simulink model "New_Wing_Monocopter_Testing"  (R2022b)
settings: Solver=ode23t  StartTime=0.0  StopTime=50  MaxStep=1e-3  RelTol=1e-3  AbsTol=1e-3
values from neighbouring files (symbols this model uses):
  air_rho = 1.225    [inherited_params.mat]
  battery_capacity = 22.8    [inherited_params.mat]
  CDO = 0.155    [inherited_params.mat]
  filtD_motor = 10000    [inherited_params.mat]
  filtSpd_motor = 0.001    [inherited_params.mat]
  kd_motor = 0    [inherited_params.mat]
  ki_motor = 0.00045    [inherited_params.mat]
  limit_motor = 0.25    [inherited_params.mat]
  monoco_mass = 0.16    [inherited_params.mat]
  monoco_prop =     [inherited_params.mat]
  monoco_radius = 0.57913    [inherited_params.mat]
  monoco_wing =     [inherited_params.mat]
  monoco_wing_area = 0.05668053    [inherited_params.mat]
  waypoints = [-2 -2 0.14 -2 -2 6 0 0 6 2 0 6 ... (15 elements, 3x5)]    [inherited_params.mat]
undefined symbols (not defined in the file or in its folder): drag_linear, drag_quad, flap_radius, flap_surface_area, klinear, kquad, X, Y, Z
libraries: sm_lib x96, nesl_utility x38, slpidlib x18, fl_lib x12, sdl_lib x3, simulink x2, simulink_extras x1, batteryecm_lib x1, ee_lib x1
(part 6 of 6)

== system New_Wing_Monocopter_Testing/Monowing/Monowing_Assem/Flap control ==
  y : Inport
  Conversion to deg : Gain  Gain=180/pi
  Conversion to rad : Gain  Gain=pi/180
  File Solid : sm_lib/Body Elements/File Solid  ExtGeomFileName=C:\Users\emman\Monocopter_Frame\DmMc_Wing_type7_Flap2.STEP  UnitType=FromFile  ExtGeomFileUnits=m  StepReaderType=HEX  ExportConvexHullGeometry=off  InertiaType=CalculateFromGeometry  Mass=0.57  MassUnits=g  CenterOfMass=[0 0 0]  CenterOfMassUnits=m  MomentsOfInertia=[1 1 1]  MomentsOfInertiaUnits=kg*m^2  ProductsOfInertia=[0 0 0]  ProductsOfInertiaUnits=kg*m^2  BasedOnType=Mass  Density=1000  DensityUnits=kg/m^3  DoExposeReferenceFrame=off  SerializedFrames=<Frames><Frame><Id>Frame1</Id><Value><Name>Flap_hinge</Name><Origin><Source>GeometricFeature</Source><FeatureName>planar surface 5</FeatureName></Origin><PrimaryAxis><DefinedDirection>+Z</DefinedDirection><Source>GeometricFeature</Source><SourceDirection>+Z</SourceDirection><FeatureName>segment 10</FeatureName></PrimaryAxis><SecondaryAxis><DefinedDirection>+X</DefinedDirection><Source>ReferenceFrame</Source><SourceDirection>+X</SourceDirection><FeatureName></FeatureName></SecondaryAxis></Value></Frame><Frame><Id>Frame2</Id><Value><Name>Flap_contact_1</Name><Origin><Source>GeometricFeature</Source><FeatureName>point 5</FeatureName></Origin><PrimaryAxis><DefinedDirection>+Z</DefinedDirection><Source>ReferenceFrame</Source><SourceDirection>+Z</SourceDirection><FeatureName></FeatureName></PrimaryAxis><SecondaryAxis><DefinedDirection>+X</DefinedDirection><Source>ReferenceFrame</Source><SourceDirection>+X</SourceDirection><FeatureName></FeatureName></SecondaryAxis></Value></Frame><Frame><Id>Frame3</Id><Value><Name>Flap_contact_2</Name><Origin><Source>GeometricFeature</Source><FeatureName>point 7</FeatureName></Origin><PrimaryAxis><DefinedDirection>+Z</DefinedDirection><Source>ReferenceFrame</Source><SourceDirection>+Z</SourceDirection><FeatureName></FeatureName></PrimaryAxis><SecondaryAxis><DefinedDirection>+X</DefinedDirection><Source>ReferenceFrame</Source><SourceDirection>+X</SourceDirection><FeatureName></FeatureName></SecondaryAxis></Value></Frame><Frame><Id>Frame4</Id><Value><Name>Flap_Moment</Name><Origin><Source>CenterOfMassFrame</Source><FeatureName></FeatureName></Origin><PrimaryAxis><DefinedDirection>+Z</DefinedDirection><Source>ReferenceFrame</Source><SourceDirection>+Z</SourceDirection><FeatureName></FeatureName></PrimaryAxis><SecondaryAxis><DefinedDirection>+X</DefinedDirection><Source>ReferenceFrame</Source><SourceDirection>+X</SourceDirection><FeatureName></FeatureName></SecondaryAxis></Value></Frame></Frames>  GraphicType=FromGeometry  MarkerShape=Sphere  MarkerSize=10  GraphicVisPropType=SimpleVisualProperties  GraphicDiffuseColor=[0.5 0.5 0.5]  GraphicSpecularColor=[0.5 0.5 0.5 1.0]  GraphicAmbientColor=[0.15 0.15 0.15 1.0]  GraphicEmissiveColor=[0.0 0.0 0.0 1.0]  GraphicShininess=75  GraphicOpacity=1.0
  PS-Simulink Converter : nesl_utility/PS-Simulink Converter  PhysicalDomain=network_engine_domain  SubClassName=ps_output  LeftPortType=input  RightPortType=output  PseudoPeriodic=off  Frequencies=[]  VectorFormat=inherit  Unit=inherit  AffineConversion=off
  Revolute Joint : sm_lib/Joints/Revolute Joint  JointMode=Normal  SenseConstraintForce=off  SenseConstraintForceX=off  SenseConstraintForceY=off  SenseConstraintForceZ=off  SenseConstraintTorque=off  SenseConstraintTorqueX=off  SenseConstraintTorqueY=off  SenseConstraintTorqueZ=off  SenseTotalForce=off  SenseTotalForceX=off  SenseTotalForceY=off  SenseTotalForceZ=off  SenseTotalTorque=off  SenseTotalTorqueX=off  SenseTotalTorqueY=off  SenseTotalTorqueZ=off  CompositeWrenchDir=FollowerOnBase  CompositeWrenchFrame=BaseFrame  EquilibriumPosition=0  EquilibriumPositionUnits=rad  SpringStiffness=0  SpringStiffnessUnits=N*m/deg  DampingCoefficient=0  DampingCoefficientUnits=N*m/(deg/s)  TorqueActuationMode=ComputedTorque  MotionActuationMode=InputMotion  SensePosition=on  SenseVelocity=off  SenseAcceleration=off  SenseTorqueForce=off  SenseLowerLimitTorqueForce=off  SenseUpperLimitTorqueForce=off  LowerLimitSpecify=off  LowerLimitBound=-20  LowerLimitBoundUnits=deg  LowerLimitStiffness=1e4  LowerLimitStiffnessUnits=N*m/deg  LowerLimitDamping=10  LowerLimitDampingUnits=N*m/(deg/s)  LowerLimitTransitionRegionWidth=0.1  LowerLimitTransitionRegionWidthUnits=deg  UpperLimitSpecify=off  UpperLimitBound=0  UpperLimitBoundUnits=deg  UpperLimitStiffness=1e4  UpperLimitStiffnessUnits=N*m/deg  UpperLimitDamping=10  UpperLimitDampingUnits=N*m/(deg/s)  UpperLimitTransitionRegionWidth=0.1  UpperLimitTransitionRegionWidthUnits=deg  PositionTargetSpecify=on  PositionTargetPriority=High  PositionTargetValue=0.0  PositionTargetValueUnits=rad  VelocityTargetSpecify=off  VelocityTargetPriority=High  VelocityTargetValue=0  VelocityTargetValueUnits=deg/s
  Rigid Transform9 : sm_lib/Frames and Transforms/Rigid Transform  TranslationMethod=Cartesian  TranslationStandardOffset=0  TranslationLengthUnit=mm  TranslationStandardAxis=+Z  TranslationCartesianOffset=[-1.5 -0.25 0.2]  TranslationROffset=0  TranslationROffsetUnits=m  TranslationZOffset=0  TranslationZOffsetUnits=m  TranslationThetaOffset=0  TranslationThetaOffsetUnits=deg  RotationMethod=None  RotationAngleUnits=deg  RotationStandardAxis=+Z  RotationAngle=0.0  RotationArbitraryAxis=[0 0 1]  FollAlignAxisA=+X  BaseAlignAxisA=+Y  FollAlignAxisB=+Y  BaseAlignAxisB=+Z  RotationSequenceAxes=FollowerAxes  RotationSequence=XYX  RotationSequenceAngles=[0 0 0]  RotationSequenceAnglesUnits=deg  RotationMatrix=[1 0 0; 0 1 0; 0 0 1]  Quaternion=[1 0 0 0]
  Simulink-PS Converter : nesl_utility/Simulink-PS Converter  PhysicalDomain=network_engine_domain  SubClassName=ps_input  LeftPortType=input  RightPortType=output  PseudoPeriodic=off  Frequencies=[]  NoiseDistribution=none  NoiseParameters=[]  Unit=rad  AffineConversion=off  FilteringAndDerivatives=filter  SimscapeFilterOrder=2  InputFilterTimeConstant=0.01  UdotUserProvided=0
  Transfer Fcn (with initial outputs) : simulink_extras/Additional Linear/Transfer Fcn (with initial outputs)  N=[1]  D="[0.01  1]"  Y0=.5  U0=0
  Conn1 : PMIOPort  Side=Left
  Flap Contact 1 : PMIOPort  Port=2  Side=Left
  Flap Contact 2 : PMIOPort  Port=3  Side=Left
  Flap Moment : PMIOPort  Port=4  Side=Left
  Out1 : Outport
  wires:
  Conversion to rad/1 -> Transfer Fcn (with initial outputs)/1
  Transfer Fcn (with initial outputs)/1 -> Simulink-PS Converter/1
  PS-Simulink Converter/1 -> Conversion to deg/1
  y/1 -> Conversion to rad/1
  Conversion to deg/1 -> Out1/1
  connections:
  Revolute Joint/RConn1 -- File Solid/LConn1
  Revolute Joint/LConn1 -- Rigid Transform9/RConn1
  Simulink-PS Converter/RConn1 -- Revolute Joint/LConn2
  PS-Simulink Converter/LConn1 -- Revolute Joint/RConn2
  Rigid Transform9/LConn1 -- Conn1/RConn1
  File Solid/RConn1 -- Flap Contact 1/RConn1
  Flap Contact 2/RConn1 -- File Solid/LConn2
  Flap Moment/RConn1 -- File Solid/RConn2

== system New_Wing_Monocopter_Testing/Collective Control/PD Alt Controller (Monoco negative direction counter clockwise)/Low Pass Filter/If Action Subsystem ==
  In1 : Inport
  Action Port : ActionPort  ActionPortLabel=else
  Out1 : Outport
  wires:
  In1/1 -> Out1/1

== system New_Wing_Monocopter_Testing/Collective Control/PD Alt Controller (Monoco negative direction counter clockwise)/Low Pass Filter/If Action Subsystem1 ==
  In1 : Inport
  Action Port : ActionPort  ActionPortLabel=if(u1<(-2200))
  Out1 : Outport
  wires:
  In1/1 -> Out1/1

== system New_Wing_Monocopter_Testing/Collective Control/PD Alt Controller (Monoco positve direction clockwise)/Low Pass Filter/If Action Subsystem ==
  In1 : Inport
  Action Port : ActionPort  ActionPortLabel=else
  Out1 : Outport
  wires:
  In1/1 -> Out1/1

== system New_Wing_Monocopter_Testing/Collective Control/PD Alt Controller (Monoco positve direction clockwise)/Low Pass Filter/If Action Subsystem1 ==
  In1 : Inport
  Action Port : ActionPort  ActionPortLabel=if(u1>(2300))
  Out1 : Outport
  wires:
  In1/1 -> Out1/1

== system New_Wing_Monocopter_Testing/Cyclic Roll Control/PD Pitch Controller (Monoco negative direction counter clockwise) Back Motor/Low Pass Filter/If Action Subsystem ==
  In1 : Inport
  Action Port : ActionPort
  Out1 : Outport
  wires:
  In1/1 -> Out1/1

== system New_Wing_Monocopter_Testing/Cyclic Roll Control/PD Pitch Controller (Monoco negative direction counter clockwise) Back Motor/Low Pass Filter/If Action Subsystem1 ==
  In1 : Inport
  Action Port : ActionPort
  Out1 : Outport
  wires:
  In1/1 -> Out1/1

== system New_Wing_Monocopter_Testing/Cyclic Roll Control/PD Pitch Controller (Monoco negative direction counter clockwise) Front Motor/Low Pass Filter/If Action Subsystem ==
  In1 : Inport
  Action Port : ActionPort
  Out1 : Outport
  wires:
  In1/1 -> Out1/1

== system New_Wing_Monocopter_Testing/Cyclic Roll Control/PD Pitch Controller (Monoco negative direction counter clockwise) Front Motor/Low Pass Filter/If Action Subsystem1 ==
  In1 : Inport
  Action Port : ActionPort
  Out1 : Outport
  wires:
  In1/1 -> Out1/1

== system New_Wing_Monocopter_Testing/Cyclic Roll Control/PD Pitch Controller (Monoco negative direction counter clockwise)2/Low Pass Filter/If Action Subsystem ==
  In1 : Inport
  Action Port : ActionPort
  Out1 : Outport
  wires:
  In1/1 -> Out1/1

== system New_Wing_Monocopter_Testing/Cyclic Roll Control/PD Pitch Controller (Monoco negative direction counter clockwise)2/Low Pass Filter/If Action Subsystem1 ==
  In1 : Inport
  Action Port : ActionPort
  Out1 : Outport
  wires:
  In1/1 -> Out1/1

== system New_Wing_Monocopter_Testing/Cyclic Roll Control/PD Roll Controller (Monoco negative direction counter clockwise) Back Motor/Low Pass Filter/If Action Subsystem ==
  In1 : Inport
  Action Port : ActionPort
  Out1 : Outport
  wires:
  In1/1 -> Out1/1

== system New_Wing_Monocopter_Testing/Cyclic Roll Control/PD Roll Controller (Monoco negative direction counter clockwise) Back Motor/Low Pass Filter/If Action Subsystem1 ==
  In1 : Inport
  Action Port : ActionPort
  Out1 : Outport
  wires:
  In1/1 -> Out1/1

== system New_Wing_Monocopter_Testing/Cyclic Roll Control/PD Roll Controller (Monoco negative direction counter clockwise) Front Motor/Low Pass Filter/If Action Subsystem ==
  In1 : Inport
  Action Port : ActionPort
  Out1 : Outport
  wires:
  In1/1 -> Out1/1

== system New_Wing_Monocopter_Testing/Cyclic Roll Control/PD Roll Controller (Monoco negative direction counter clockwise) Front Motor/Low Pass Filter/If Action Subsystem1 ==
  In1 : Inport
  Action Port : ActionPort
  Out1 : Outport
  wires:
  In1/1 -> Out1/1

== matlab function New_Wing_Monocopter_Testing/Monowing/Speed Brake mode/Speed Brake Mode Activation ==
  data: rps input; y output; monoco_radius parameter; pitch input; air_rho parameter; monoco_wing_area parameter; Time input; Mode input
function y = fcn(rps, monoco_radius, pitch, air_rho, monoco_wing_area, Time, Mode)
linear_vel_sq = zeros(1,1);
linear_vel_sq = (rps * monoco_radius)^2;
drag_angle = 120;
drag_coeff = 0.1;



if Mode == 0
    if (pitch > drag_angle) && (Time < 8.0) 
        y = 0.5 * drag_coeff * air_rho * monoco_wing_area * linear_vel_sq * monoco_radius;
    else
        y = 0.0;
    end
else
    y = 0.0;
end

== matlab function New_Wing_Monocopter_Testing/Monowing/Collective Control/Collective (Anhedral) ==
  data: Torque_negative input; Toggle input; output output
function output  = fcn(Torque_negative, Toggle)

if Toggle == 2.0
    output = Torque_negative * 1.0; % change this 
else
    output = 0.0;
end
%y = Torque_negative;

== matlab function New_Wing_Monocopter_Testing/Monowing/Drag State/Drag filter ==
  data: drag input; Time input; drag_upper output; drag_lower output; Mode input
function [drag_upper, drag_lower] = fcn(drag, Time, Mode)
if Mode == 0
    if Time > 8.0 && Time < 12.0
        drag_upper = drag;
        drag_lower = 0.0;
    elseif Time > 12.0
        drag_lower = -1 * drag;
        drag_upper = 0.0;
    else
        drag_upper = drag;
        drag_lower = 0.0;
    end

elseif Mode == 1
    drag_upper = drag;
    drag_lower = 0.0;

else
    drag_upper = 0.0;
    drag_lower = -1 * drag;

end

== matlab function New_Wing_Monocopter_Testing/Hover ==
  data: Y output; toggle_y output; X output; toggle_x output; Time input
function [Y, toggle_y, X, toggle_x] = fcn(Time)

sol_X = zeros(1,1);
sol_Toggle_Y = zeros(1,1);
sol_Toggle_X = zeros(1,1);
sol_Y = zeros(1,1);
Velocity = 0.2;

if Time > 10 && Time < 40
%     if Time > 10 && Time < 15
%         sol_X = 0;
%         sol_Toggle_Y = 1;
%         sol_Toggle_X = 1;
%         sol_Y = -1;
%     
%     elseif Time > 15 && Time < 20
%         sol_X = 0;
%         sol_Toggle_Y = 1;
%         sol_Toggle_X = 1;
%         sol_Y = 0;
%     
%     elseif Time > 20 && Time < 25
%         sol_X = 0;
%         sol_Toggle_Y = 1;
%         sol_Toggle_X = 1;
%         sol_Y = 1;
% 
%     elseif Time > 25 && Time < 30
%         sol_X = 0;
%         sol_Toggle_Y = 1;
%         sol_Toggle_X = 1;
%         sol_Y = 0;
%     end
% 
% else
    sol_X = 0;
    sol_Y = 0;
    sol_Toggle_Y = 1;
    sol_Toggle_X = 1;
end

Y = sol_Y;
X = sol_X;
toggle_y = sol_Toggle_Y;
toggle_x = sol_Toggle_X;

== matlab function New_Wing_Monocopter_Testing/Monowing/Monowing_Assem/Collective & Cyclic Command Distribution (Dihedral Pitch) abt Yw ==
  data: u input; flap_dihedral_pitch_cmd output; gain_x input; heading input; Toggle input; Motor_Pulse output
function [flap_dihedral_pitch_cmd,Motor_Pulse] = fcn(u, gain_x, heading, Toggle)

if Toggle == 1 % Front Motor

    azimuth = u;
    if (abs(azimuth) > pi/4) && (abs(azimuth) < 3*pi/4)
        tilt_xw = sin(azimuth + heading); % tilt about yw heading in x direction 
        pitch = zeros(1,1);
        pitch = tilt_xw * gain_x; % only for cyclic y
        Motor_Pulse =  (pitch/abs(pitch)) * 1;

        if abs(pitch) > 0.75
            pitch = (pitch/abs(pitch)) * 0.75;
        end

        flap_dihedral_pitch_cmd = pitch;

    else
        
        Motor_Pulse =  0;
        flap_dihedral_pitch_cmd = 0.0;

    end

elseif Toggle == 2 % Back Motor

    azimuth = u;
    if (abs(azimuth) > pi/4) && (abs(azimuth) < 3*pi/4)
        tilt_xw = sin(azimuth + heading); % tilt around xw heading in y direction 
        pitch = zeros(1,1);
        pitch = tilt_xw * gain_x; % only for cyclic y
        Motor_Pulse =  (pitch/abs(pitch)) * 1;

        if abs(pitch) > 0.75
            pitch = (pitch/abs(pitch)) * 0.75;
        end

        flap_dihedral_pitch_cmd = pitch;

    else
        
        Motor_Pulse =  0;
        flap_dihedral_pitch_cmd = 0.0;

    end

else
    
    Motor_Pulse =  0;
    flap_dihedral_pitch_cmd = 0.0;

end





% kp = 1.3;
% desired_roll = 10;
% if (Annular_roll/abs(Annular_roll)) > 0.0
%     error_gain = kp*(Annular_roll - desired_roll);
% 
% elseif (Annular_roll/abs(Annular_roll)) < 0.0
%     error_gain = kp*(Annular_roll - (-1*desired_roll));
% 
% else
%     error_gain = 0.0;
% 
% end

% roll = gain * desired_flap * 2; % only for cyclic (original) 
% roll = desired_flap; % collective
% flap_cmd = roll - error_gain;

== matlab function New_Wing_Monocopter_Testing/Monowing/Monowing_Assem/Cyclic Command Distribution ==
  data: pitch_gain_dihedral_front input; roll_gain_dihedral_front input; pitch_gain_dihedral_back input; roll_gain_dihedral_back input; Transition_Mode output; gain_x output; gain_y output; Dihedral_Mode output; Mode_Selection input
function [Transition_Mode, gain_x, gain_y, Dihedral_Mode] = fcn(pitch_gain_dihedral_front, roll_gain_dihedral_front, pitch_gain_dihedral_back, roll_gain_dihedral_back, Mode_Selection)

if Mode_Selection == 1
    Transition_Mode = 0;
    Dihedral_Mode = 1;
    gain_x = pitch_gain_dihedral_front;
    gain_y = roll_gain_dihedral_front;
else 
    Transition_Mode = 0;
    Dihedral_Mode = 2;
    gain_x = pitch_gain_dihedral_back;
    gain_y = roll_gain_dihedral_back;
end



% if Mode_Selection == 0
%     Transition_Mode = 1;
%     Dihedral_Mode = 0;
%     Anhedral_Mode = 0;
%     gain_x = 0;
%     gain_y = 0;
% elseif Mode_Selection == 1
%     Transition_Mode = 0;
%     Dihedral_Mode = 1;
%     Anhedral_Mode = 0;
%     gain_x = pitch_gain_dihedral;
%     gain_y = roll_gain_dihedral;
% elseif Mode_Selection == 2
%     Transition_Mode = 0;
%     Dihedral_Mode = 0;
%     Anhedral_Mode = 1;
%     gain_x = pitch_gain_anhedral;
%     gain_y = roll_gain_anhedral;
% else 
%     Transition_Mode = 0;
%     Dihedral_Mode = 0;
%     Anhedral_Mode = 0;
%     gain_x = 0;
%     gain_y = 0;
% end

== matlab function New_Wing_Monocopter_Testing/Monowing/Collective Control/Collective Mode Switcher ==
  data: dihedral output; Time input; anhedral output; Mode input
function [dihedral,anhedral] = fcn(Time,Mode)
if Mode == 1
      dihedral = 1.0;
      anhedral = 0.0;
    
elseif Mode == 2
    dihedral = 1.0;
    anhedral = 0.0;
else
    dihedral = 0.0;
    anhedral = 0.0;
end


% if Mode == 0
%     
%     if Time > 8.0 && Time < 12.0
%         dihedral = 0.0; % upside cut torque
%         anhedral = 0.0;
%     elseif Time > 10
%         dihedral = 0.0;
%         anhedral = 1.0;
%     else
%         dihedral = 1.0;
%         anhedral = 0.0;
%     end
% 
% elseif Mode == 1
% 
%     dihedral = 1.0;
%     anhedral = 0.0;
% 
% elseif Mode == 2
% 
%     dihedral = 0.0;
%     anhedral = 1.0;
% 
% else
% 
%     dihedral = 0.0;
%     anhedral = 0.0;
% 
% end

== matlab function New_Wing_Monocopter_Testing/Monowing/Horizontal Forces/Horizontal Motion X ==
  data: roll_in_deg input; force output; Lift input; flap_angle_data input; vx input; vy input; vz input; klinear parameter; kquad parameter; pos_x input; azimuth input; flap_angle input
function force  = fcn(roll_in_deg, Lift, flap_angle_data, vx, vy, vz, klinear, kquad, pos_x, azimuth, flap_angle)
fx = zeros(1,1);
x = zeros(1,1);
v_l1 = zeros(1,1);
v_l2 = zeros(1,1);
roll_angle = abs(roll_in_deg);
%disp(Lift);
dihedral_offset = 2.0;
v_l1 = abs(vx) + abs(vy) + abs(vz);
v_l2 = sqrt(vx^2 + vy^2 + vz^2);

negative_x = 0;
positive_x = 1;
neutral_x = 2;

if azimuth > 0 && flap_angle > 0 
    current_state = negative_x;
    
elseif azimuth < 0 && flap_angle < 0
    current_state = negative_x;

elseif azimuth > 0 && flap_angle < 0
    current_state = positive_x;

elseif azimuth < 0 && flap_angle > 0
    current_state = positive_x;

else
    current_state = neutral_x;
end

%disp (current_state);
% disp (azimuth);
% disp (flap_angle);

% current_state = negative_y;

switch(current_state)

    case negative_x
        if roll_in_deg > 0 && roll_in_deg > dihedral_offset 
        %     if roll_in_deg > 0
            fx = Lift*sind(roll_in_deg-dihedral_offset);
            x = (-1*fx) + (kquad*v_l1*abs(vy) + klinear*abs(vy));
        elseif roll_in_deg < 0
            fx = Lift*sind(roll_angle);
            x = (-1*fx) + (kquad*v_l1*abs(vy) + klinear*abs(vy));
            %y = y  (kquad*v_l1*abs(vy) + klinear*abs(vy));
        else
            x = 0.0;
        end

    case positive_x
        if roll_in_deg > 0 && roll_in_deg > dihedral_offset 
        %     if roll_in_deg > 0
            fx = Lift*sind(roll_in_deg-dihedral_offset);
            x = fx - (kquad*v_l1*abs(vy) + klinear*abs(vy));
        elseif roll_in_deg < 0
            fx = Lift*sind(roll_angle);
            x = fx - (kquad*v_l1*abs(vy) + klinear*abs(vy));
            %y = y  (kquad*v_l1*abs(vy) + klinear*abs(vy));
        else
            x = 0.0;
        end

    case neutral_x 
            x = 0.0;

end

force = x;
% Acceleration_in_x_axis = x/monoco_mass;
% flap_angle_recording = flap_angle_data;

== matlab function New_Wing_Monocopter_Testing/Monowing/Monowing_Assem/Collective & Cyclic Command Distribution (Dihedral Roll) abt Xw ==
  data: u input; flap_dihedral_roll_cmd output; gain_y input; heading input; Toggle input; Motor_Pulse output
function [flap_dihedral_roll_cmd,Motor_Pulse] = fcn(u, gain_y, heading, Toggle)

if Toggle == 1 % Front Motor

    azimuth = u;
    if (abs(azimuth) > 3*pi/4) || (abs(azimuth) < pi/4)
        tilt_yw = cos(azimuth + heading); % tilt around xw heading in y direction 
        roll = zeros(1,1);
        roll = tilt_yw * gain_y; % only for cyclic y
        Motor_Pulse =  (roll/abs(roll)) * 1;

        if abs(roll) > 0.6
            roll = (roll/abs(roll)) * 0.6;
        end

        flap_dihedral_roll_cmd = roll;

    else
        
        Motor_Pulse =  0;
        flap_dihedral_roll_cmd = 0.0;

    end

elseif Toggle == 2 % Back Motor

    azimuth = u;
    if (abs(azimuth) > 3*pi/4) || (abs(azimuth) < pi/4)
        tilt_yw = cos(azimuth + heading); % tilt around xw heading in y direction 
        roll = zeros(1,1);
        roll = tilt_yw * gain_y; % only for cyclic y
        Motor_Pulse =  (roll/abs(roll)) * 1;

        if abs(roll) > 0.6
            roll = (roll/abs(roll)) * 0.6;
        end

        flap_dihedral_roll_cmd = roll;

    else
        
        Motor_Pulse =  0;
        flap_dihedral_roll_cmd = 0.0;

    end

else
    
    Motor_Pulse =  0;
    flap_dihedral_roll_cmd = 0.0;

end







% kp = 1.3;
% desired_roll = 10;
% if (Annular_roll/abs(Annular_roll)) > 0.0
%     error_gain = kp*(Annular_roll - desired_roll);
% 
% elseif (Annular_roll/abs(Annular_roll)) < 0.0
%     error_gain = kp*(Annular_roll - (-1*desired_roll));
% 
% else
%     error_gain = 0.0;
% 
% end

% roll = gain * desired_flap * 2; % only for cyclic (original) 
% roll = desired_flap; % collective
% flap_cmd = roll - error_gain;

== matlab function New_Wing_Monocopter_Testing/Cyclic Roll Control/PD Roll Controller (Monoco negative direction counter clockwise) Front Motor/Gain Switching ==
  data: aggro input; y output; Toggle input; annular_roll input; gentle input
function y = fcn(aggro, Toggle, annular_roll, gentle)

if Toggle > 0
    if abs(annular_roll) > 5.0
        y = aggro;
    else
        y = gentle;
    end
else
    y = 0;
end

% y = gentle;

== matlab function New_Wing_Monocopter_Testing/Motor speed 2 motor induced torque plot (Back Motor) ==
  data: u input; y output; Mode input
function y = fcn(u, Mode)
coder.extrinsic('fit');
input = u;

%disp (size(u));

%%%%% generate motor torque %%%%%%%%%%
% speed = [-8414 -11985 -13823 -15490 -16851 -18122 -19334 -20546 -21868 -23218 -24568 -25568 -26403 -27239 -28264 -29297 -30294 -31211 -31578 0 8414 11985 13823 15490 16851 18122 19334 20546 21868 23218 24568 25568 26403 27239 28264 29297 30294 31211 31578];
% %speed = transpose(speed);
% power = [-14.88 -21.18 -31 -41.67 -53.85 -66.98 -80.75 -94.53 -110.53 -127.1 -143.66 -161.84 -180.78 -199.72 -213.16 -226.38 -243.4 -268.51 -279.30 0 14.88 21.18 31 41.67 53.85 66.98 80.75 94.53 110.53 127.1 143.66 161.84 180.78 199.72 213.16 226.38 243.4 268.51 279.30];
% %power = transpose(power);
% torque = mrdivide(power,speed);
% %torque = transpose(torque);
% disp(torque);

% f = fit(speed,torque,'poly3'); % speed torque function
% disp (f);
% disp (f(-10));
% plot(f,speed,torque);
% xlabel('RPM')
% ylabel('Torque')
% title('Motor plot torque vs speed')


% conversion2rpm = 0.10471975513824;
% x = abs(input)/conversion2rpm; 
if Mode == 2
    y = 0.0031 * -1;  % dun change!
else
    y = 0.0031 * 0;
end
 
    
% y = 0.0066 * 0;

%y= 0;
% disp("func is");
% disp(y);
% disp("input is");
% disp(input);

== matlab function New_Wing_Monocopter_Testing/Diamond ==
  data: Y output; toggle_y output; X output; toggle_x output; Time input; Z output
function [Y, toggle_y, X, toggle_x, Z] = fcn(Time)

sol_X = zeros(1,1);
sol_Toggle_Y = zeros(1,1);
sol_Toggle_X = zeros(1,1);
sol_Y = zeros(1,1);
Velocity = 0.35;

z = 2.3; 
if Time > 10 && Time < 37
    if Time > 10 && Time < 16
        sol_X = -2;
        sol_Toggle_Y = 1;
        sol_Toggle_X = 1;
        sol_Y = 2;
        z = 2.3; 
    
    elseif Time > 16 && Time < 27
        sol_X = 2;
        sol_Toggle_Y = 1;
        sol_Toggle_X = 1;
        sol_Y = 2;
        z = 2.0; 
    
    elseif Time > 27 && Time < 33
        sol_X = 0;
        sol_Toggle_Y = 1;
        sol_Toggle_X = 1;
        sol_Y = 0;
        z = 2.0; 
    end

else
    sol_X = 0;
    sol_Y = 0;
    sol_Toggle_Y = 0;
    sol_Toggle_X = 0;
end

Y = sol_Y;
X = sol_X;
Z = z;
toggle_y = sol_Toggle_Y;
toggle_x = sol_Toggle_X;

== matlab function New_Wing_Monocopter_Testing/Square Trajectory ==
  data: Y output; toggle_y output; X output; toggle_x output; Time input
function [Y, toggle_y, X, toggle_x] = fcn(Time)

sol_X = zeros(1,1);
sol_Toggle_Y = zeros(1,1);
sol_Toggle_X = zeros(1,1);
sol_Y = zeros(1,1);
Velocity = 0.2;

if Time > 6 && Time < 120
    if Time > 6 && Time < 16
        sol_X = 2;
        sol_Toggle_Y = 1;
        sol_Toggle_X = 1;
        sol_Y = 0;
    
    elseif Time > 16 && Time < 26
        sol_X = 2;
        sol_Toggle_Y = 1;
        sol_Toggle_X = 1;
        sol_Y = 4;
    
    elseif Time > 26 && Time < 36
        sol_X = -2;
        sol_Toggle_Y = 1;
        sol_Toggle_X = 1;
        sol_Y = 4;
    
    elseif Time > 32 && Time < 42
        sol_X = -2;
        sol_Toggle_Y = 1;
        sol_Toggle_X = 1;
        sol_Y = 0;
    
    elseif Time > 42 && Time < 50
        sol_X = 0;
        sol_Toggle_Y = 1;
        sol_Toggle_X = 1;
        sol_Y = 0;
    end

else
    sol_X = 0;
    sol_Y = 0;
    sol_Toggle_Y = 0;
    sol_Toggle_X = 0;
end

Y = sol_Y;
X = sol_X;
toggle_y = sol_Toggle_Y;
toggle_x = sol_Toggle_X;

== matlab function New_Wing_Monocopter_Testing/Monowing/flap_moment  ==
  data: flap_angle input; y output; rps input; monoco_radius parameter; air_rho parameter; flap_surface_area parameter; flap_radius parameter
function y = fcn(flap_angle, rps, monoco_radius, air_rho, flap_surface_area, flap_radius)
linear_vel_sq = zeros(1,1);
linear_vel_sq = (rps * monoco_radius)^2;
y = flap_radius * 0.5 * 0.005 * flap_angle * air_rho * flap_surface_area * linear_vel_sq;

== matlab function New_Wing_Monocopter_Testing/Motor speed 2 motor induced torque plot (Front Motor) ==
  data: u input; y output; Mode input
function y = fcn(u, Mode)
coder.extrinsic('fit');
input = u;

%disp (size(u));

%%%%% generate motor plot %%%%%%%%%%
% speed = [-8414 -11985 -13823 -15490 -16851 -18122 -19334 -20546 -21868 -23218 -24568 -25568 -26403 -27239 -28264 -29297 -30294 -31211 -31578 0 8414 11985 13823 15490 16851 18122 19334 20546 21868 23218 24568 25568 26403 27239 28264 29297 30294 31211 31578];
% %speed = transpose(speed);
% power = [-14.88 -21.18 -31 -41.67 -53.85 -66.98 -80.75 -94.53 -110.53 -127.1 -143.66 -161.84 -180.78 -199.72 -213.16 -226.38 -243.4 -268.51 -279.30 0 14.88 21.18 31 41.67 53.85 66.98 80.75 94.53 110.53 127.1 143.66 161.84 180.78 199.72 213.16 226.38 243.4 268.51 279.30];
% %power = transpose(power);
% torque = mrdivide(power,speed);
% %torque = transpose(torque);
% disp(torque);

% f = fit(speed,torque,'poly3'); % speed torque function
% disp (f);
% disp (f(-10));
% plot(f,speed,torque);
% xlabel('RPM')
% ylabel('Torque')
% title('Motor plot torque vs speed')


% conversion2rpm = 0.10471975513824;
% x = abs(input)/conversion2rpm; 
if Mode == 1
    y = 0.0031 * 1; % dun change!
else
    %y = 0.0066 * 0;
    y = 0.0031 * 0; 
end    
% y = 0.0066 * 0;

%y= 0;
% disp("func is");
% disp(y);
% disp("input is");
% disp(input);

== matlab function New_Wing_Monocopter_Testing/Cyclic Roll Control/PD Pitch Controller (Monoco negative direction counter clockwise) Front Motor/Gain Switching2 ==
  data: aggro input; y output; Toggle input; annular_roll input; gentle input
function y = fcn(aggro, Toggle, annular_roll, gentle)

if Toggle > 0
    if abs(annular_roll) > 5.0
        y = aggro;
    else
        y = gentle;
    end
else
    y = 0;
end


% y = gentle;

== matlab function New_Wing_Monocopter_Testing/Collective Control/PD Alt Controller (Monoco negative direction counter clockwise)/Motor Pulsing Filter ==
  data: u input; y output; toggle input
function y = fcn(u, toggle)

motor_pulse = zeros(1,1);

if toggle == 1
    motor_pulse = -1 * abs(u);
elseif toggle == -1
    motor_pulse = abs(u);
else
    motor_pulse = 0;
end

if abs(motor_pulse) > 300
    motor_pulse = motor_pulse/abs(motor_pulse) * 300;

end

y = motor_pulse;

== matlab function New_Wing_Monocopter_Testing/Y Test ==
  data: Y output; toggle_y output; X output; toggle_x output; Time input
function [Y, toggle_y, X, toggle_x] = fcn(Time)

sol_X = zeros(1,1);
sol_Toggle_Y = zeros(1,1);
sol_Toggle_X = zeros(1,1);
sol_Y = zeros(1,1);
Velocity = 0.2;

if Time > 10 && Time < 40
%     if Time > 10 && Time < 15
%         sol_X = 0;
%         sol_Toggle_Y = 1;
%         sol_Toggle_X = 1;
%         sol_Y = -1;
%     
%     elseif Time > 15 && Time < 20
%         sol_X = 0;
%         sol_Toggle_Y = 1;
%         sol_Toggle_X = 1;
%         sol_Y = 0;
%     
%     elseif Time > 20 && Time < 25
%         sol_X = 0;
%         sol_Toggle_Y = 1;
%         sol_Toggle_X = 1;
%         sol_Y = 1;
% 
%     elseif Time > 25 && Time < 30
%         sol_X = 0;
%         sol_Toggle_Y = 1;
%         sol_Toggle_X = 1;
%         sol_Y = 0;
%     end
% 
% else
    sol_X = 0;
    sol_Y = 0;
    sol_Toggle_Y = 1;
    sol_Toggle_X = 1;
end

Y = sol_Y;
X = sol_X;
toggle_y = sol_Toggle_Y;
toggle_x = sol_Toggle_X;

== matlab function New_Wing_Monocopter_Testing/X Test ==
  data: Y output; toggle_y output; X output; toggle_x output; Time input
function [Y, toggle_y, X, toggle_x] = fcn(Time)

sol_X = zeros(1,1);
sol_Toggle_Y = zeros(1,1);
sol_Toggle_X = zeros(1,1);
sol_Y = zeros(1,1);
Velocity = 0.2;

if Time > 10 && Time < 40
    if Time > 10 && Time < 18
        sol_X = -2;
        sol_Toggle_Y = 0;
        sol_Toggle_X = 1;
        sol_Y = 0;
    
    elseif Time > 18 && Time < 30
        sol_X = 2;
        sol_Toggle_Y = 0;
        sol_Toggle_X = 1;
        sol_Y = 0;
    
    elseif Time > 30 && Time < 40
        sol_X = 0;
        sol_Toggle_Y = 0;
        sol_Toggle_X = 1;
        sol_Y = 0;
    end

else
    sol_X = 0;
    sol_Y = 0;
    sol_Toggle_Y = 0;
    sol_Toggle_X = 0;
end

Y = sol_Y;
X = sol_X;
toggle_y = sol_Toggle_Y;
toggle_x = sol_Toggle_X;

== matlab function New_Wing_Monocopter_Testing/Collective Control/PD Alt Controller (Monoco negative direction counter clockwise)/Motor speed 2 thrust plot ==
  data: u input; y output
function y = fcn(u)
coder.extrinsic('fit');
input = u;

%disp (size(u));

%%%%% generate motor plot %%%%%%%%%%
% conversion2rads = 0.10471975513824;
% convert2Newton = 9.81/1000; 
% speed = conversion2rads.*[-31578 -31211 -30294 -29297 -28264 -27239 -26403 -25568 -24568 -23218 -21868 -20546 -19344 -18122 -16851 -15490 -13823 -11985 -8414 0 8414 11985 13823 15490 16851 18122 19334 20546 21868 23218 24568 25568 26403 27239 28264 29297 30294 31211 31578];
% speed = transpose(speed);
% thrust = convert2Newton.*[-485,-475,-450,-425,-400,-375,-350,-325,-300,-275,-250,-225,-200,-175,-150,-125,-100,-75,-50,0,50,75,100,125,150,175,200,225,250,275,300,325,350,375,400,425,450,475,485];
% thrust = transpose(thrust);
% f = fit(speed,thrust,'poly3'); % speed thrust function
% disp (f);
% disp (f(-10));
% plot(f,speed,thrust);
% xlabel('RPS')
% ylabel('Force')
% title('Motor plot force vs speed')

% rps = (100/2290).*[2290 2175.5 2061 1946.5 1832 1717.5 1603 1488.5 1374 1259.5 1145 1030.5 916];
% rps = transpose(rps);
% rot_freq = 0.1591549.*[30.2 28.82 27.5 26.21 24.95 23.71 22.5 21.3 20.13 18.97 17.82 16.67 15.5];
% rot_freq = transpose(rot_freq);
% g = fit(rps,rot_freq,'poly2');  % high thrust = high rotational freq = high lift
% disp(g);
% plot(g,rps,rot_freq);
% xlabel('thrust(%)')
% ylabel('rot_freq(hz)')
% title('thrust vs rot_freq')


x = input; 
% prev % func = 7.884e-11*x^3 - 7.663e-12*x^2 + 0.0006131*x + 8.695e-05; % motor speed(rps) vs thrust(N) ~ approximation, this value is the approx motor thrust obtained from motor rps
func = 4.975e-11*x^3 + 3.747e-23*x^2 + 0.0003889*x - 3.142e-16;
y = func;


%y= 0;
% disp("func is");
% disp(y);
% disp("input is");
% disp(input);

== matlab function New_Wing_Monocopter_Testing/Cyclic Roll Control/PD Roll Controller (Monoco negative direction counter clockwise) Back Motor/Gain Switching ==
  data: aggro input; y output; Toggle input; annular_roll input; gentle input
function y = fcn(aggro, Toggle, annular_roll, gentle)

if Toggle > 0
    if abs(annular_roll) > 5
        y = aggro;
    else
        y = gentle;
    end
else
    y = 0;
end

% y = gentle;

== matlab function New_Wing_Monocopter_Testing/Cyclic Roll Control/PD Pitch Controller (Monoco negative direction counter clockwise)2/Gain Switching2 ==
  data: aggro input; y output; Toggle input; annular_roll input; gentle input
function y = fcn(aggro, Toggle, annular_roll, gentle)

if Toggle > 0
    if abs(annular_roll) < 2.75
        y = aggro;
    else
        y = gentle;
    end
else
    y = 0;
end

== matlab function New_Wing_Monocopter_Testing/Cyclic Roll Control/PD Pitch Controller (Monoco negative direction counter clockwise) Back Motor/Gain Switching2 ==
  data: aggro input; y output; Toggle input; annular_roll input; gentle input
function y = fcn(aggro, Toggle, annular_roll, gentle)

if Toggle > 0
    if abs(annular_roll) > 5.0
        y = aggro;
    else
        y = gentle;
    end
else
    y = 0;
end

% y = gentle;

== matlab function New_Wing_Monocopter_Testing/Monowing/Quat2Eul Function ==
  data: u input; Euler_Angles_Collectively output size=[1 4] [-1000..1000]; bod_pitch_deg_abt_Xb output size=[1,1]; bod_roll_deg_abt_Yb output; body_yaw_rad_z output; Pos output size=[1 5]; Time input; pos_x input; pos_y input; pos_z input; rps input
function [Euler_Angles_Collectively, bod_pitch_deg_abt_Xb, bod_roll_deg_abt_Yb, body_yaw_rad_z, Pos] = fcn(u, Time, pos_x, pos_y, pos_z, rps)
coder.extrinsic('quat2eul');
anx = zeros(1,3);
body_pitch_deg = zeros(1,1);
body_roll_deg = zeros(1,1);
yaw_rad = zeros(1,1);
quat = flip(transpose(u));
% disp (quat);

eul = quat2eul(quat); % ZYX 
% Z = zeros(1,1);

% Body frame dynamics
Z = eul(1,1);
Y = eul(1,2);
X = eul(1,3);
body_pitch_deg = rad2deg(X);
body_roll_deg = rad2deg(Y);
% yaw_deg = rad2deg(Z);
yaw_rad = Z;

anx = rad2deg([X Y Z]);
Pos = [Time pos_x pos_y pos_z rps];
% disp (size(deg));
% disp (size(Z));
Euler_Angles_Collectively = [Time, anx];

% World frame dynamics
% annular_pitch_deg_abt_yw = -1*body_pitch_deg; % anti clockwise is negative but i negate it so its easier to read; annular y axis in world frame
% annular_roll_deg_abt_xw = 1*body_roll_deg; % clockwise is positive; annular x axis in world frame

% Body frame dynamics
bod_pitch_deg_abt_Xb = -1*body_pitch_deg;
bod_roll_deg_abt_Yb = 1*body_roll_deg;
body_yaw_rad_z = yaw_rad;

== matlab function New_Wing_Monocopter_Testing/Monowing/Monowing_Assem/Collective & Cyclic Command Distribution (Transition) ==
  data: stalling_flap input; flap_transition_cmd output; Time input; Toggle input
function flap_transition_cmd = fcn(stalling_flap,Time, Toggle)
if Toggle == 1
    
    roll = zeros(1,1);
    roll = stalling_flap; % collective
    
    if Time > 8.0
        flap_transition_cmd = 0.0;
    else 
        flap_transition_cmd = roll;
    end

else

    flap_transition_cmd = 0.0;

end

== matlab function New_Wing_Monocopter_Testing/Monowing/Drag moment/Drag Moment (X & Y) ==
  data: y input; drag_moment_abt_y output; drag_linear parameter; drag_quad parameter; x input; drag_moment_abt_x output; azimuth input
function [drag_moment_abt_y,drag_moment_abt_x] = fcn(y, drag_linear, drag_quad, x, azimuth)
drag_moment_y  = zeros(1,1);
drag_moment_x  = zeros(1,1);
gain = cos(azimuth);
drag_moment_y = (drag_linear * y) + (drag_quad * y^2); 
drag_moment_x = (drag_linear * x) + (drag_quad * x^2); 

drag_moment_abt_y = -1 * drag_moment_y;
drag_moment_abt_x = -1 * drag_moment_x;

== matlab function New_Wing_Monocopter_Testing/Monowing/Horizontal Forces/Horizontal Motion Y ==
  data: roll_in_deg input; force output; Lift input; flap_angle_data input; flap_angle_recording output; vx input; vy input; vz input; klinear parameter; kquad parameter; pos_y input; azimuth input; flap_angle input
function [force, flap_angle_recording] = fcn(roll_in_deg, Lift, flap_angle_data, vx, vy, vz, klinear, kquad, pos_y, azimuth, flap_angle)
fy = zeros(1,1);
y = zeros(1,1);
v_l1 = zeros(1,1);
v_l2 = zeros(1,1);
roll_angle = abs(roll_in_deg);
%disp(Lift);
dihedral_offset = 2.0;
v_l1 = abs(vx) + abs(vy) + abs(vz);
v_l2 = sqrt(vx^2 + vy^2 + vz^2);

negative_y = 0;
positive_y = 1;
neutral_y = 2;

if abs(azimuth) < pi/2 && flap_angle > 0 
    current_state = negative_y;
    
elseif abs(azimuth) > pi/2 && flap_angle < 0
    current_state = negative_y;

elseif abs(azimuth) > pi/2 && flap_angle > 0
    current_state = positive_y;

elseif abs(azimuth) < pi/2 && flap_angle < 0
    current_state = positive_y;

else
    current_state = neutral_y;
end

% disp (current_state);
% disp (azimuth);
% disp (flap_angle);

% current_state = negative_y;

switch(current_state)

    case negative_y
        if roll_in_deg > 0 && roll_in_deg > dihedral_offset 
        %     if roll_in_deg > 0
            fy = Lift*sind(roll_in_deg-dihedral_offset);
            y = (-1*fy) + (kquad*v_l1*abs(vy) + klinear*abs(vy));
        elseif roll_in_deg < 0
            fy = Lift*sind(roll_angle);
            y = (-1*fy) + (kquad*v_l1*abs(vy) + klinear*abs(vy));
            %y = y  (kquad*v_l1*abs(vy) + klinear*abs(vy));
        else
            y = 0.0;
        end

    case positive_y
        if roll_in_deg > 0 && roll_in_deg > dihedral_offset 
        %     if roll_in_deg > 0
            fy = Lift*sind(roll_in_deg-dihedral_offset);
            y = fy - (kquad*v_l1*abs(vy) + klinear*abs(vy));
        elseif roll_in_deg < 0
            fy = Lift*sind(roll_angle);
            y = fy - (kquad*v_l1*abs(vy) + klinear*abs(vy));
            %y = y  (kquad*v_l1*abs(vy) + klinear*abs(vy));
        else
            y = 0.0;
        end

    case neutral_y 
            y = 0.0;

end

force = y;
% Acceleration_in_y_axis = y/monoco_mass;
flap_angle_recording = flap_angle_data;

== matlab function New_Wing_Monocopter_Testing/Monowing/Collective Control/Collective (Dihedral) ==
  data: Torque_negative input; output output; Toggle input
function output  = fcn(Torque_negative,Toggle)

if Toggle == 1 
    output = Torque_negative;
else
    output = 0;
end

== matlab function New_Wing_Monocopter_Testing/Collective Control/PD Alt Controller (Monoco positve direction clockwise)/Motor speed 2 thrust plot ==
  data: u input; y output
function y = fcn(u)
coder.extrinsic('fit');
input = u;

%disp (size(u));

%%%%% generate motor plot %%%%%%%%%%
% conversion2rads = 0.10471975513824;
% convert2Newton = 9.81/1000; 
% speed = conversion2rads.*[-31578 -31211 -30294 -29297 -28264 -27239 -26403 -25568 -24568 -23218 -21868 -20546 -19344 -18122 -16851 -15490 -13823 -11985 -8414 0 8414 11985 13823 15490 16851 18122 19334 20546 21868 23218 24568 25568 26403 27239 28264 29297 30294 31211 31578];
% speed = transpose(speed);
% thrust = convert2Newton.*[-485,-475,-450,-425,-400,-375,-350,-325,-300,-275,-250,-225,-200,-175,-150,-125,-100,-75,-50,0,50,75,100,125,150,175,200,225,250,275,300,325,350,375,400,425,450,475,485];
% thrust = transpose(thrust);
% f = fit(speed,thrust,'poly3'); % speed thrust function
% disp (f);
% disp (f(-10));
% plot(f,speed,thrust);
% xlabel('RPS')
% ylabel('Force')
% title('Motor plot force vs speed')

% rps = (100/2290).*[2290 2175.5 2061 1946.5 1832 1717.5 1603 1488.5 1374 1259.5 1145 1030.5 916];
% rps = transpose(rps);
% rot_freq = 0.1591549.*[30.2 28.82 27.5 26.21 24.95 23.71 22.5 21.3 20.13 18.97 17.82 16.67 15.5];
% rot_freq = transpose(rot_freq);
% g = fit(rps,rot_freq,'poly2');  % high thrust = high rotational freq = high lift
% disp(g);
% plot(g,rps,rot_freq);
% xlabel('thrust(%)')
% ylabel('rot_freq(hz)')
% title('thrust vs rot_freq')


x = input; 
func = 7.884e-11*x^3 - 7.663e-12*x^2 + 0.0006131*x + 8.695e-05; % motor speed(rps) vs thrust(N) ~ approximation, this value is the approx motor thrust obtained from motor rps 
y = func;


%y= 0;
% disp("func is");
% disp(y);
% disp("input is");
% disp(input);
